simulink model "NonUniformQuantificationVoice"  (R2018b)
settings: Solver=VariableStepAuto  StartTime=0.0  StopTime=10.0  RelTol=1e-3
undefined symbols (not defined in the file): ln, sgn, xmax
settings Model: Creator=Anderson  LastModifiedBy=Anderson

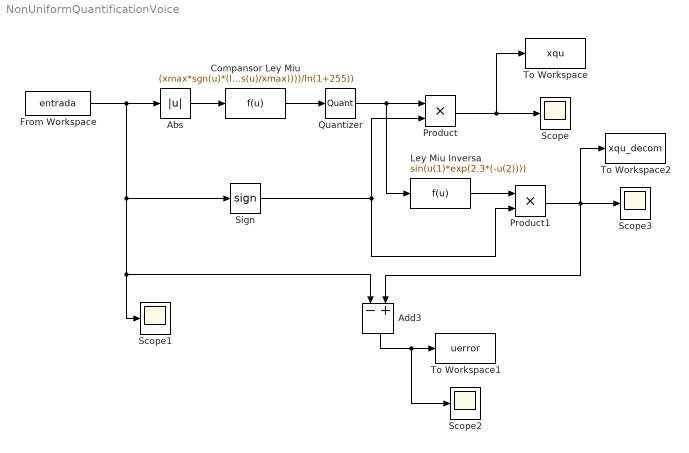
== system NonUniformQuantificationVoice ==
  Abs : Abs
  Add3 : Sum  Inputs=-+
  Compansor Ley Miu : Fcn  Expr=(xmax*sgn(u)*(ln(1+(255*(abs(u)/xmax))))/ln(1+255))
  From Workspace : FromWorkspace  VariableName=entrada  SampleTime=0
  Ley Miu Inversa : Fcn  Expr=sin(u(1)*exp(2.3*(-u(2))))
  Product : Product
  Product1 : Product
  Quantizer : Quantizer  QuantizationInterval=0.125
  Scope{,1..3} (4 alike) : Scope
  Sign : Signum
  To Workspace : ToWorkspace  VariableName=xqu  SaveFormat=Timeseries  SampleTime=-1
  To Workspace1 : ToWorkspace  VariableName=uerror  SaveFormat=Timeseries  SampleTime=-1
  To Workspace2 : ToWorkspace  VariableName=xqu_decom  SaveFormat=Timeseries  SampleTime=-1
  wires:
  From Workspace/1 -> Abs/1, Add3/1, Scope1/1, Sign/1
  Add3/1 -> Scope2/1, To Workspace1/1
  Abs/1 -> Compansor Ley Miu/1
  Compansor Ley Miu/1 -> Quantizer/1
  Quantizer/1 -> Ley Miu Inversa/1, Product/1
  Ley Miu Inversa/1 -> Product1/1
  Sign/1 -> Product1/2, Product/2
  Product/1 -> To Workspace/1, Scope/1
  Product1/1 -> Add3/2, To Workspace2/1, Scope3/1
